simulink model "warehouseTasksRobot"  (R2020b)
settings: Solver=FixedStepAuto  StartTime=0.0  StopTime=inf  FixedStep=0.1  RelTol=1e-3
values from neighbouring files (symbols this model uses):
  chargingStn = [90 50]    [modelInitial.mat]
  loadingStn = [58 21]    [modelInitial.mat]
  logicalMap = [1 1 1 1 1 1 1 1 1 1 1 1 ... (10000 elements, 100x100)]    [modelInitial.mat]
  logicalMapObs = logical(mmp)    [createObs.m]    (also in example.m = createObs(logicalMap, obstacle, influate_size); modelInitial.mat = [1 1 1 1 1 1 1 1 1 1 1 1 ... (10000 elements, 100x100)])
  obstacle = [35 30]    [modelInitial.mat]
  unloadingStn = [20 58]    [modelInitial.mat]
libraries: robotalgslib x2, robotmobilelib x1
settings Model: Creator=fan  LastModifiedBy=fan

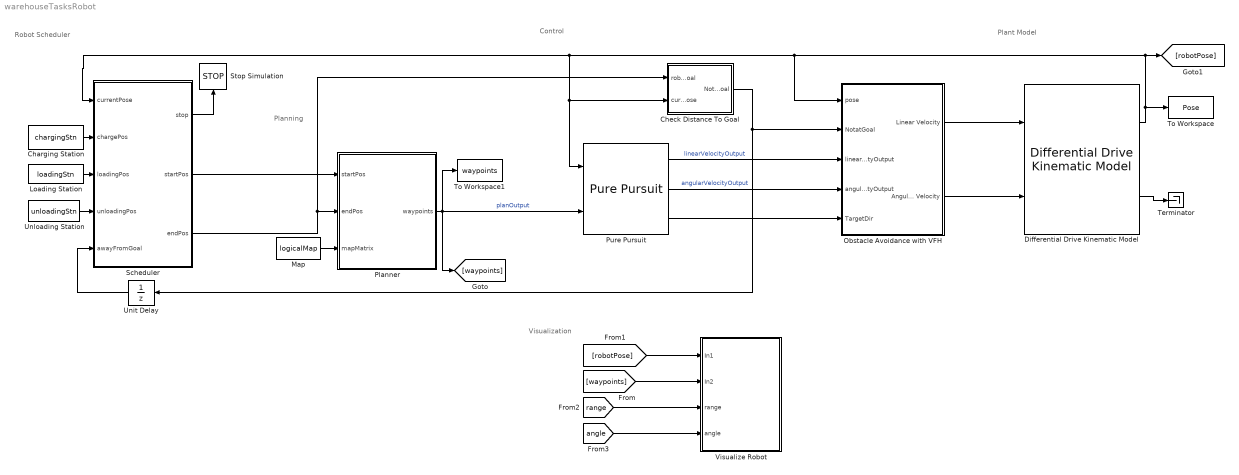
== system warehouseTasksRobot ==
  note: Plant Model
  note: Planning
  note: Control
  note: Robot Scheduler
  note: Visualization
  "Charging Station " : Constant  Value=chargingStn  SampleTime=1
  Check Distance To Goal : Subsystem
  "Differential Drive Kinematic Model " : robotmobilelib/Differential Drive Kinematic Model  VehicleInputs=Vehicle Speed & Heading Angular Velocity  WheelRadius=0.1  WheelSpeedRange=[-inf inf]  TrackWidth=0.3  InitialState=[chargingStn,0]'  SimulateUsing=Code generation
      settings: SourceProductName=Robotics System Toolbox
  Loading Station : Constant  Value=loadingStn
  "Map " : Constant  Value=logicalMap  SampleTime=1
  Obstacle Avoidance with VFH : Subsystem
  Planner : MATLAB Function  TreatAsAtomicUnit=on
  Pure Pursuit : robotalgslib/Pure Pursuit  DesiredLinearVelocity=0.1  MaxAngularVelocity=1.0  LookaheadDistance=0.5  TargetDirPort=on  SimulateUsing=Code generation
  Scheduler : Stateflow chart  TreatAsAtomicUnit=on
  Stop Simulation : Stop
  Terminator : Terminator
  To Workspace : ToWorkspace  VariableName=Pose  SampleTime=-1
  To Workspace1 : ToWorkspace  VariableName=waypoints  SampleTime=-1
  Unit Delay : UnitDelay  SampleTime=-1  HasFrameUpgradeWarning=on
  Unloading Station : Constant  Value=unloadingStn  SampleTime=1
  Visualize Robot : Subsystem  mask{MeshSelectionIdx=Ground vehicle, PresetViews=Entire Map, ShowViz=on, ShowPaths=on, MapXMin=0, MapXMax=100, MapYMin=0, MapYMax=100, XLimits=[0 size(logicalMap, 1)], YLimits=[0 size(logicalMap, 2)], LocalXLimits=[-10 10], LocalYLimits=[-10 10], ChargingLocation=chargingStn, SortingStation=loadingStn, UnloadingStation=unloadingStn, ObstacleLocation=obstacle, VisualizationSampleRate=5}
      mask prompts: MeshSelectionIdx "Robot mesh"; PresetViews "Preset Views"; ShowViz "Update visualization:"; ShowPaths "Show planned paths:"; MapXMin "Map xmin:"; MapXMax "Map xmax:"; MapYMin "Map ymin:"; MapYMax "Map ymax:"; XLimits "Map x-limits:"; YLimits "Map y-limits:"; LocalXLimits "Local view x-limits"; LocalYLimits "Local view y-limits"; ChargingLocation "Start locations:"; SortingStation "Dock locations:"; UnloadingStation "Shelf locations:"; ObstacleLocation "Obstacle locations:"; VisualizationSampleRate "Sample time:"
      mask init:
      | % Create the list of key locations
      | startLocationMatrix = evalin('base', get_param(gcb, 'ChargingLocation'));
      | shelfLocationMatrix = evalin('base', get_param(gcb, 'UnloadingStation'));
      | dockLocationMatrix = evalin('base', get_param(gcb, 'SortingStation'));
      | 
      | % Create popup list from matrices
      | dockLocationNameCell = cell(size(dockLocationMatrix,1),1);
      | shelfLocationNameCell = cell(size(shelfLocationMatrix,1),1);
      | startLocationNameCell = cell(size(startLocationMatrix,1),1);
      | for i = 1:size(startLocationMatrix,1)
      |     startLocationNameCell{i} = ['Charging Station ' num2str(i)];
      | end
      | for j = 1:size(shelfLocationMatrix,1)
      |     shelfLocationNameCell{j} = ['Unloading Station ' num2str(j)];
      | end
      | for k = 1:size(dockLocationMatrix,1)
      |     dockLocationNameCell{k} = ['Sorting Station ' num2str(k)];
      | end
      | 
      | % Update the parameter list
      | m = Simulink.Mask.get(gcb);
      | viewPopupParam = m.getParameter('PresetViews');
      | viewPopupParam.TypeOptions = [...
      |     {'Entire Map'}; ...
      |     dockLocationNameCell; ...
      |     shelfLocationNameCell; ...
      |     startLocationNameCell ... 
      |     ];
      mask TypeOptions MeshSelectionIdx: Ground vehicle | Forklift
      mask TypeOptions PresetViews: Entire Map | Sorting Station 1 | Unloading Station 1 | Charging Station 1
      mask Callback PresetViews:
      | % Get key numeric data
      | startLocationMatrix = evalin('base', get_param(gcb, 'ChargingLocation'));
      | dockLocationMatrix = evalin('base', get_param(gcb, 'SortingStation'));
      | shelfLocationMatrix = evalin('base', get_param(gcb, 'UnloadingStation'));
      | mapXLim = evalin('base', get_param(gcb, 'XLimits'));
      | mapYLim = evalin('base', get_param(gcb, 'YLimits'));
      | viewXLim = evalin('base', get_param(gcb, 'LocalXLimits'));
      | viewYLim = evalin('base', get_param(gcb, 'LocalYLimits'));
      | 
      | % Get selected value
      | viewSelection = get_param(gcb, 'PresetViews');
      | 
      | %Take action based on view
      | if strcmp(viewSelection, 'Custom')
      |     % Do nothing
      | else
      |     if strcmp(viewSelection(1:5), 'Charg')
      |         % Start location
      |         startIndex = str2double(viewSelection(end));
      |         localPts = startLocationMatrix(startIndex, :);
      |         viewLimits = [localPts(1)+viewXLim(1) localPts(1)+viewXLim(2) ...
      |             localPts(2)+viewYLim(1) localPts(2)+viewYLim(2)];
      | 
      |     elseif strcmp(viewSelection(1:5), 'Sorti')
      |         % Dock (Loading) location
      |         dockIndex = str2double(viewSelection(end));
      |         localPts = dockLocationMatrix(dockIndex, :);
      |         viewLimits = [localPts(1)+viewXLim(1) localPts(1)+viewXLim(2) ...
      |             localPts(2)+viewYLim(1) localPts(2)+viewYLim(2)];
      | 
      |     elseif strcmp(viewSelection(1:5), 'Unloa')
      |         % Shelf (Unloading) location
      |         shelfIndex = str2double(viewSelection(end));
      |         localPts = shelfLocationMatrix(shelfIndex, :);
      |         viewLimits = [localPts(1)+viewXLim(1) localPts(1)+viewXLim(2) ...
      |             localPts(2)+viewYLim(1) localPts(2)+viewYLim(2)];
      | 
      |     else
      |         % Show the whole map
      |         viewLimits = [mapXLim(1) mapXLim(2) mapYLim(1) mapYLim(2)];
      |     end
      | 
      |     % Set the map parameters
      |     set_param(gcb, 'MapXMin', num2str(viewLimits(1)));
      |     set_param(gcb, 'MapXMax', num2str(viewLimits(2)));
      |     set_param(gcb, 'MapYMin', num2str(viewLimits(3)));
      |     set_param(gcb, 'MapYMax', num2str(viewLimits(4)));
      | end
      mask Callback MapXMin:
      | currentMax = str2num(get_param(gcb, 'MapXMax'));
      | newMin = str2num(get_param(gcb, 'MapXMin'));
      | if newMin > currentMax
      |     set_param(gcb, 'MapXMax', num2str(newMin+1));
      | end
      mask Callback MapXMax:
      | currentMin = str2num(get_param(gcb, 'MapXMin'));
      | newMax = str2num(get_param(gcb, 'MapXMax'));
      | if newMax < currentMin
      |     set_param(gcb, 'MapXMin', num2str(newMax-1));
      | end
      mask Callback MapYMin:
      | currentMax = str2num(get_param(gcb, 'MapYMax'));
      | newMin = str2num(get_param(gcb, 'MapYMin'));
      | if newMin > currentMax
      |     set_param(gcb, 'MapYMax', num2str(newMin+1));
      | end
      mask Callback MapYMax:
      | currentMin = str2num(get_param(gcb, 'MapYMin'));
      | newMax = str2num(get_param(gcb, 'MapYMax'));
      | if newMax < currentMin
      |     set_param(gcb, 'MapYMin', num2str(newMax-1));
      | end
      mask DialogControl DescGroupVar Prompt: Visualization example helper
      mask DialogControl DescTextVar Prompt: This subsystem plots the robots and environement and allows users to change the views.
      mask DialogControl ViewLimits Prompt: View limits
      mask DialogControl ViewConfigurationGroup Prompt: View configuration:
      mask DialogControl ViewParamSourcesGroup Prompt: View parameter sources
      mask Display: disp('Visualization Helper')
  wires:
  Obstacle Avoidance with VFH/2(Angular Velocity) -> "Differential Drive Kinematic Model "/2
  Scheduler/3(endPos) -> Check Distance To Goal/1(robotGoal), Planner/2(endPos)
  Unloading Station/1 -> Scheduler/4(unloadingPos)
  [waypoints] -> Visualize Robot/2(In2)
  Pure Pursuit/1 -> Obstacle Avoidance with VFH/3(linearVelocityOutput)  "linearVelocityOutput"
  Scheduler/1(stop) -> Stop Simulation/1
  Unit Delay/1 -> Scheduler/5(awayFromGoal)
  "Charging Station "/1 -> Scheduler/2(chargePos)
  "Map "/1 -> Planner/3(mapMatrix)
  Check Distance To Goal/1(NotatGoal) -> Unit Delay/1, Obstacle Avoidance with VFH/2(NotatGoal)
  "Differential Drive Kinematic Model "/2 -> Terminator/1
  Planner/1(waypoints) -> Pure Pursuit/2, To Workspace1/1, [waypoints]  "planOutput"
  [robotPose] -> Visualize Robot/1(In1)
  [range] -> Visualize Robot/3(range)
  Loading Station/1 -> Scheduler/3(loadingPos)
  [angle] -> Visualize Robot/4(angle)
  Obstacle Avoidance with VFH/1(Linear Velocity) -> "Differential Drive Kinematic Model "/1
  Pure Pursuit/3 -> Obstacle Avoidance with VFH/5(TargetDir)
  "Differential Drive Kinematic Model "/1 -> [robotPose], Obstacle Avoidance with VFH/1(pose), Check Distance To Goal/2(currentPose), Pure Pursuit/1, Scheduler/1(currentPose), To Workspace/1
  Pure Pursuit/2 -> Obstacle Avoidance with VFH/4(angularVelocityOutput)  "angularVelocityOutput"
  Scheduler/2(startPos) -> Planner/1(startPos)

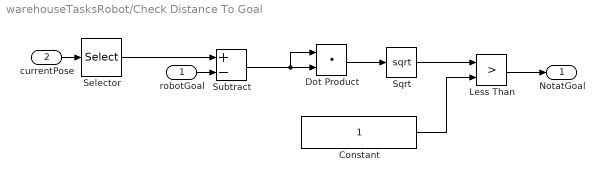
== system warehouseTasksRobot/Check Distance To Goal ==
  robotGoal : Inport
  currentPose : Inport  Port=2
  Constant : Constant
  Dot Product : DotProduct  InputSameDT=on  OutDataTypeStr=Inherit: Inherit via internal rule
  Less Than : RelationalOperator  Operator=>  OutDataTypeStr=boolean  RndMeth=Simplest
  Selector : Selector  InputPortWidth=3  IndexOptions=Index vector (dialog)  Indices=[1 2]  OutputSizes=1
  Sqrt : Sqrt  SaturateOnIntegerOverflow=on
  Subtract : Sum  Inputs=+-
  NotatGoal : Outport
  wires:
  robotGoal/1 -> Subtract/2
  Dot Product/1 -> Sqrt/1
  Constant/1 -> Less Than/2
  currentPose/1 -> Selector/1
  Less Than/1 -> NotatGoal/1
  Sqrt/1 -> Less Than/1
  Subtract/1 -> Dot Product/1, Dot Product/2
  Selector/1 -> Subtract/1

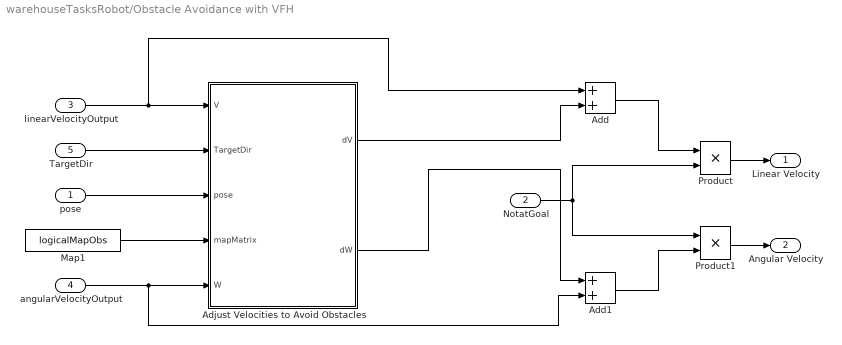
== system warehouseTasksRobot/Obstacle Avoidance with VFH ==
  pose : Inport
  NotatGoal : Inport  Port=2
  linearVelocityOutput : Inport  Port=3
  angularVelocityOutput : Inport  Port=4
  TargetDir : Inport  Port=5
  Add : Sum
  Add1 : Sum
  Adjust Velocities to Avoid Obstacles : Subsystem
  Map1 : Constant  Value=logicalMapObs
  Product : Product
  Product1 : Product
  Linear Velocity : Outport  OutDataTypeStr=double
  Angular Velocity : Outport  Port=2  OutDataTypeStr=double
  wires:
  NotatGoal/1 -> Product/2, Product1/1
  Product/1 -> Linear Velocity/1
  Product1/1 -> Angular Velocity/1
  Adjust Velocities to Avoid Obstacles/2(dW) -> Add1/1
  angularVelocityOutput/1 -> Adjust Velocities to Avoid Obstacles/5(W), Add1/2
  Add1/1 -> Product1/2
  Add/1 -> Product/1
  Map1/1 -> Adjust Velocities to Avoid Obstacles/4(mapMatrix)
  linearVelocityOutput/1 -> Add/1, Adjust Velocities to Avoid Obstacles/1(V)
  Adjust Velocities to Avoid Obstacles/1(dV) -> Add/2
  TargetDir/1 -> Adjust Velocities to Avoid Obstacles/2(TargetDir)
  pose/1 -> Adjust Velocities to Avoid Obstacles/3(pose)

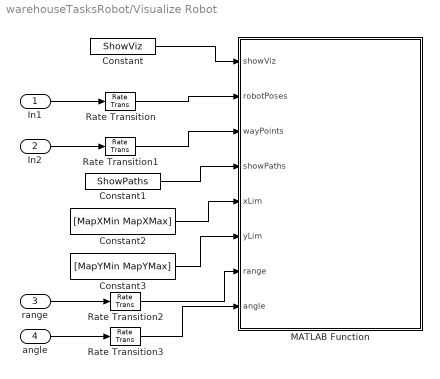
== system warehouseTasksRobot/Visualize Robot ==
  In1 : Inport
  In2 : Inport  Port=2
  range : Inport  Port=3
  angle : Inport  Port=4
  Constant : Constant  Value=ShowViz
  Constant1 : Constant  Value=ShowPaths
  Constant2 : Constant  Value=[MapXMin MapXMax]
  Constant3 : Constant  Value=[MapYMin MapYMax]
  MATLAB Function : MATLAB Function  TreatAsAtomicUnit=on
  Rate Transition{,1..3} (4 alike) : RateTransition
  wires:
  In2/1 -> Rate Transition1/1
  In1/1 -> Rate Transition/1
  Rate Transition/1 -> MATLAB Function/2(robotPoses)
  Rate Transition1/1 -> MATLAB Function/3(wayPoints)
  Constant/1 -> MATLAB Function/1(showViz)
  Constant1/1 -> MATLAB Function/4(showPaths)
  Constant2/1 -> MATLAB Function/5(xLim)
  Constant3/1 -> MATLAB Function/6(yLim)
  range/1 -> Rate Transition2/1
  Rate Transition2/1 -> MATLAB Function/7(range)
  angle/1 -> Rate Transition3/1
  Rate Transition3/1 -> MATLAB Function/8(angle)

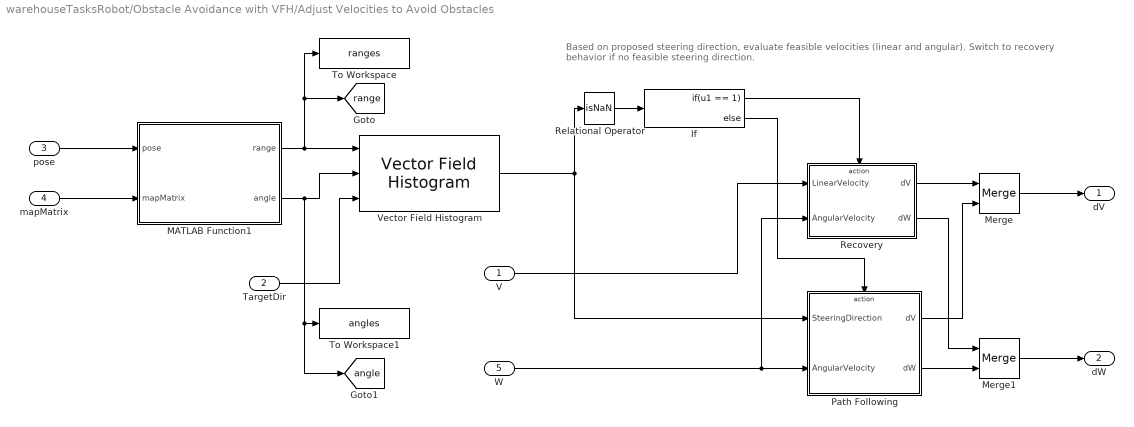
== system warehouseTasksRobot/Obstacle Avoidance with VFH/Adjust Velocities to Avoid Obstacles ==
  note: Based on proposed steering direction, evaluate feasible velocities (linear and angular).
      | 				Switch to recovery behavior if no feasible steering direction.
  V : Inport
  TargetDir : Inport  Port=2
  pose : Inport  Port=3
  mapMatrix : Inport  Port=4
  W : Inport  Port=5
  If : If  IfExpression=u1 == 1
  MATLAB Function1 : MATLAB Function  TreatAsAtomicUnit=on
  Merge : Merge
  Merge1 : Merge
  Path Following : Subsystem  TreatAsAtomicUnit=on
  Recovery : Subsystem  TreatAsAtomicUnit=on
  Relational Operator : RelationalOperator  Operator=isNaN  OutDataTypeStr=boolean  RndMeth=Simplest
  To Workspace : ToWorkspace  VariableName=ranges  SampleTime=-1
  To Workspace1 : ToWorkspace  VariableName=angles  SampleTime=-1
  Vector Field Histogram : robotalgslib/Vector Field Histogram  NumAngularSectors=180  DistanceLimits=[ 0.05, 3 ]  HistogramThresholds=[ 3, 8 ]  RobotRadius=0.5  SafetyDistance=0.6  MinTurningRadius=0.5  SimulateUsing=Code generation  TargetDirectionWeight=5  CurrentDirectionWeight=2  PreviousDirectionWeight=2
      settings: SourceProductBaseCode=NV,RO
  dV : Outport  VectorParamsAs1DForOutWhenUnconnected=off
  dW : Outport  Port=2  VectorParamsAs1DForOutWhenUnconnected=off
  tag scope: angle=global, range=global
  wires:
  Merge1/1 -> dW/1
  V/1 -> Recovery/1(LinearVelocity)
  W/1 -> Recovery/2(AngularVelocity), Path Following/2(AngularVelocity)
  Relational Operator/1 -> If/1
  Merge/1 -> dV/1
  If/1 -> Recovery/Action
  If/2 -> Path Following/Action
  Recovery/2(dW) -> Merge1/1
  Path Following/2(dW) -> Merge1/2
  Recovery/1(dV) -> Merge/1
  Path Following/1(dV) -> Merge/2
  pose/1 -> MATLAB Function1/1(pose)
  mapMatrix/1 -> MATLAB Function1/2(mapMatrix)
  Vector Field Histogram/1 -> Path Following/1(SteeringDirection), Relational Operator/1
  MATLAB Function1/1(range) -> [range], To Workspace/1, Vector Field Histogram/1
  MATLAB Function1/2(angle) -> [angle], To Workspace1/1, Vector Field Histogram/2
  TargetDir/1 -> Vector Field Histogram/3

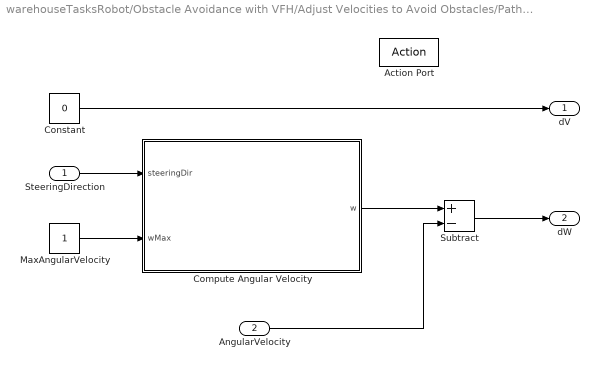
== system warehouseTasksRobot/Obstacle Avoidance with VFH/Adjust Velocities to Avoid Obstacles/Path Following ==
  SteeringDirection : Inport
  AngularVelocity : Inport  Port=2
  Action Port : ActionPort  ActionPortLabel=else
  Compute Angular Velocity : MATLAB Function  TreatAsAtomicUnit=on
  Constant : Constant  Value=0
  MaxAngularVelocity : Constant
  Subtract : Sum  Inputs=+-
  dV : Outport  VectorParamsAs1DForOutWhenUnconnected=off
  dW : Outport  Port=2  VectorParamsAs1DForOutWhenUnconnected=off
  wires:
  Constant/1 -> dV/1
  MaxAngularVelocity/1 -> Compute Angular Velocity/2(wMax)
  SteeringDirection/1 -> Compute Angular Velocity/1(steeringDir)
  Subtract/1 -> dW/1
  Compute Angular Velocity/1(w) -> Subtract/1
  AngularVelocity/1 -> Subtract/2

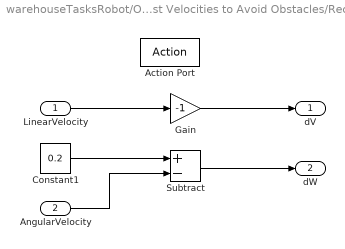
== system warehouseTasksRobot/Obstacle Avoidance with VFH/Adjust Velocities to Avoid Obstacles/Recovery ==
  LinearVelocity : Inport
  AngularVelocity : Inport  Port=2
  Action Port : ActionPort  ActionPortLabel=if(u1 == 1)
  Constant1 : Constant  Value=0.2
  Gain : Gain  Gain=-1
  Subtract : Sum  Inputs=+-
  dV : Outport  VectorParamsAs1DForOutWhenUnconnected=off
  dW : Outport  Port=2  VectorParamsAs1DForOutWhenUnconnected=off
  wires:
  LinearVelocity/1 -> Gain/1
  Gain/1 -> dV/1
  Constant1/1 -> Subtract/1
  AngularVelocity/1 -> Subtract/2
  Subtract/1 -> dW/1

== matlab function warehouseTasksRobot/Planner ==
  settings: updateMethod=DISCRETE
  data: startPos input size=[1 2]; endPos input size=[1 2]; waypoints output size=[100 2]; mapMatrix input
function waypoints = planning(startPos, endPos, mapMatrix)

persistent waypointsInternal
persistent prevStartPos
persistent prevEndPos

% Set constant parameters
maxNumNodes = 100;

% Initialize persistent variables that are used downstream
if isempty(prevStartPos)
    prevStartPos = startPos;
end

if isempty(prevEndPos)
    prevEndPos = endPos;
end

isNewPath = (~isequal(prevStartPos, startPos) || ~isequal(prevEndPos, endPos));

if isempty(waypointsInternal) || isNewPath
    % Two conditions in which waypoints must be set: they are not yet
    % initialized, or they are initialized, but the current start and end
    % do not match those used to generate the previous set of waypoints
    [waypointsInternal] = planPath(mapMatrix, maxNumNodes, startPos, endPos);
end

% Update the outputs
waypoints = waypointsInternal;

% Update the persistent variables that indicate previous state
prevStartPos = startPos;
prevEndPos = endPos;

%% Helper Function

function wayPoints = planPath(mapMatrix, maxNodes, startPos, endPos)
    
    % Create a probabilistic roadmap
    map = binaryOccupancyMap(mapMatrix);
    prm = mobileRobotPRM(map, 500);
    
    % Find a path between two points
    xy = findpath(prm, startPos(:)', endPos(:)');
    wayPoints = repmat(endPos(:)', maxNodes, 1);
    
    % Number of nodes that are actually used
    numNodes = length(xy);
    wayPoints(1:numNodes,:) = xy;    

end

end

== matlab function warehouseTasksRobot/Visualize Robot/MATLAB Function ==
  settings: updateMethod=DISCRETE  sampleTime=VisualizationSampleRate
  data: showViz input; robotPoses input; wayPoints input; logicalMapObs parameter; ChargingLocation parameter; UnloadingStation parameter; SortingStation parameter; showPaths input; xLim input; yLim input; MeshSelectionIdx parameter; range input; angle input; ObstacleLocation parameter
function simulationVisualization(showViz, robotPoses, wayPoints, logicalMapObs, ChargingLocation, UnloadingStation, SortingStation, showPaths, xLim, yLim, MeshSelectionIdx, range, angle, ObstacleLocation)
%#codegen

%% Setup

coder.extrinsic('VisualizeExecuteRobots');
persistent f
if isempty(f) && showViz
    f = figure('units','normalized','outerposition',[0 0 0.75 0.75]);
    title('Mobile Robot Motion');
    set(f, 'Visible', 'on');
end

% Robot mesh options are cells of the unloaded and loaded robot mesh and
% the translation between the visualized origin and the desired origin
meshOptions = {...
    {'groundvehicle.stl', [.314 0 .155], 'groundvehiclewithload.stl', [.312 0 .156]}, ...
    {'forkliftExecuteRobotTasks.stl', [.3569 0 .297], 'forkliftwithload.stl', [.3813 0 .2893]}, ...
    };
    

if showViz && ~isempty(f)
    VisualizeExecuteRobots(f, robotPoses, wayPoints, logicalMapObs, ChargingLocation, UnloadingStation, SortingStation, ObstacleLocation, showPaths, xLim, yLim, meshOptions{MeshSelectionIdx}, range, angle);
end
end

== stateflow chart warehouseTasksRobot/Scheduler ==
  settings: sampleTime=0.01
  state Unloading
    entry, during:
    endPos = unloadingPos';
  state Loading
    entry,during:
    endPos = loadingPos';
  state Charging
    entry, during:
    endPos = chargePos';
  (default) -> Loading : {startPos = chargePos';}
  Loading -> Unloading : [~awayFromGoal && after(stopDelay, tick)]
      |
      | {startPos = currentPose(1:2)';}
  Unloading -> Charging : [~awayFromGoal  && after(stopDelay, tick)]
      | {startPos = currentPose(1:2)';}
  Charging -> (junction 201) : [~awayFromGoal]{stop = 1;}
  data: currentPose input; stop output =0; chargePos input size=[2 1]; loadingPos input size=[2 1]; unloadingPos input size=[2 1]; startPos output size=[1, 2]; endPos output size=[1, 2]; awayFromGoal input; stopDelay local =0.7e4

== matlab function warehouseTasksRobot/Obstacle Avoidance with VFH/Adjust Velocities to Avoid Obstacles/MATLAB Function1 ==
  settings: updateMethod=DISCRETE
  data: range output; pose input size=[3, 1]; mapMatrix input; angle output
function [range, angle]  = RangeSensor(pose, mapMatrix)
persistent r
if isempty(r)
 r = rangeSensor('HorizontalAngle', [-pi/2, pi/2], 'HorizontalAngleResolution', pi/20, 'Range', [0 12]);
end
[range, angle] = r(pose', binaryOccupancyMap(mapMatrix, 1));


end

== matlab function warehouseTasksRobot/Obstacle Avoidance with VFH/Adjust Velocities to Avoid Obstacles/Path Following/Compute Angular Velocity ==
  data: steeringDir input; w output; wMax input
function w = ComputeAngularVelocity(steeringDir, wMax)

% Allow variable input arguments
if nargin == 1   
    wMax = inf;
end

validateattributes(steeringDir, {'double'},{'real'},...
    'exampleHelperComputeAngularVelocity', 'STEERINGDIR', 1);
validateattributes(wMax, {'double'},{'real', 'positive'},...
    'exampleHelperComputeAngularVelocity', 'WMAX', 2);

% Computing in robot's coordinate frame
curPose = [0 0 0];

% The following computation is similar to robotics.PurePursuit
lookaheadPoint = [cos(steeringDir), sin(steeringDir)];
slope = atan2((lookaheadPoint(2) - curPose(2)), ...
    (lookaheadPoint(1) - curPose(1)));
alpha = angdiff(curPose(3), slope);

% Angular velocity command for a differential drive robot is
% equal to the desired curvature to be followed by the robot.

w = (2*sin(alpha));

% Pick a constant rotation when robot is facing in the opposite
% direction of the path
if abs(abs(alpha) - pi) < 1e-12
    w = sign(w)*1;
end

if abs(w) > wMax
    w = sign(w)*wMax;
end

end
